simulink model "sldemo_fuelsys"  (R2022a)
settings: Solver=ode45  StartTime=0  StopTime=2000  FixedStep=0.001  RelTol=1e-5  AbsTol=1e-6
PostLoadFcn:
  | sldemo_fuelsys_data(bdroot,'initialize_data','orig','float');
model workspace (MAT data in the model file):
  PressEst = [0.806253176324 0.553142316929 0.37151500209 0.277667903103 0.220198954207 0.181288665766 0.153200000489 0.115431020872 0.0913067476324 0.0746519188607 0.0625231108324 0.0533383634277 ... (306 elements, 18x17)]
  PressVect = [0.05 0.1 0.15 0.2 0.25 0.3 0.35 0.4 0.45 0.5 0.55 0.6 0.65 0.7 0.75 0.8 0.85 0.9 0.95]
  PumpCon = [-0.0556348 -0.0022828 0.0256932 0.0435188 0.0562692 0.0661194857143 0.0741572 0.08697 0.0972452 0.106070342857 0.1139892 0.121303866667 ... (342 elements, 18x19)]
  RampRateKiX = [100 200 300 400 500 600]
  RampRateKiY = [0 0.2 0.4 0.6 0.8 1]
  RampRateKiZ = [0.012  0.024  0.036  0.048  0.06  0.072; 0.024  0.048  0.072  0.096  0.12  0.144; 0.036  0.072  0.108  0.144  0.18  0.216; 0.048  0.096  0.144  0.192  0.24  0.288; 0.06  0.12  0.18  0.24  0.3  0.36; 0.072  0.144  0.216  0.288  0.36  0.432]
  SpeedEst = [471.837839721 550.80940091 777.559313277 1080.9243499 1418.36795322 1769.7468768 2125.37309264 2480.20345067 2831.37796793 3177.14006959 3516.32917143 4064.90417867 ... (323 elements, 17x19)]
  SpeedVect = [50 75 100 125 150 175 200 250 300 350 400 450 500 600 700 800 900 1000]
  ThrotEst = [0 0 0 0 0 0 0 0 0 0 0 0 ... (342 elements, 18x19)]
  ThrotVect = [0 3 6 9 12 15 18 21 24 27 30 35 46 57 68 79 90]
  ego_sw = 1
  engine_speed = 300
  hys = 25
  map_sw = 1
  max_ego = 1.2
  max_press = 0.95
  max_speed = 628
  max_throt = 90
  min_press = 0.05
  min_speed = 50
  min_throt = 3
  speed_sw = 1
  st_range = 0.0001
  throttle_sw = 1
  zero_thresh = 250
undefined symbols (not defined in the file or in its folder): DiscIntNeverNeededParam, sld_FuelModes, sldvsubsys
libraries: simulink x4, simulink_extras x1
(part 1 of 2)
CloseFcn:
  | clear EngSensors u8En* s16En* sldemo_fuelsys_output
Description:
  | This is a model of a fuel control system where Stateflow(R) is used to handle the fault management of the system.
  | The system contains four separate sensors: a throttle sensor, a speed sensor, an oxygen sensor, and a pressure sensor.
  | Each of these sensors is represented by a parallel state in Stateflow.  Each parallel state contains two substates, a
  | normal state and a failed state (the exception being the oxygen sensor, which also contains a warmup state).
  | 
  | If any of the sensor readings is outside an acceptable range, then a fault is registered in Stateflow, and the
  | substate of the corresponding subsystem transitions to the failed state.  If a subsystem recovers, it can
  | transition back to the normal state.  The number of failures in the system at any given time is represented
  | in the Fail parallel state.
  | 
  | The last parallel state in the Stateflow chart is called Fueling_Mode.  This state regulates the oxygen to
  | fuel mixture ratio.  If a failure is detected, then the oxygen to fuel ratio is increased.  If multiple failures
  | are detected, then the fuel system is disabled until there are no longer multiple failures in the system.
settings Model: ModifiedByFormat=The MathWorks Inc.  ExtModeTrigMode=oneshot  ExtModeArmWhenConnect=off  Creator=The MathWorks, Inc.  LastModifiedBy=The MathWorks Inc.
settings SolverCC: AutoScaleAbsTol=off  AlgebraicLoopSolver=TrustRegion  MaxZcPerStep=1
settings DataIOCC: SaveFormat=StructureWithTime  SaveOutput=off  SaveTime=off  ReturnWorkspaceOutputs=off  SignalLoggingName=sldemo_fuelsys_output
settings OptimizationCC: DefaultParameterBehavior=Inlined  UseDivisionForNetSlopeComputation=UseDivisionForReciprocalsOfIntegersOnly  InlineInvariantSignals=on  EnhancedBackFolding=on  StrengthReduction=on  BooleansAsBitfields=on  PassReuseOutputArgsAs=Individual arguments  ExpressionDepthLimit=2147483647  ZeroExternalMemoryAtStartup=off  ZeroInternalMemoryAtStartup=off  NoFixptDivByZeroProtection=on  EfficientFloat2IntCast=on  LifeSpan=1  EfficientTunableParamExpr=on
settings DebuggingCC: SignalInfNanChecking=error  SaveWithParameterizedLinksMsg=none  UnderspecifiedInitializationDetection=Classic  CheckExecutionContextPreStartOutputMsg=on  IntegerOverflowMsg=none  ParameterDowncastMsg=warning  ParameterOverflowMsg=none  ParameterPrecisionLossMsg=none  UnderSpecifiedDataTypeMsg=warning  FcnCallInpInsideContextMsg=warning  UnconnectedInputMsg=warning  UnconnectedOutputMsg=warning  UnconnectedLineMsg=warning  UniqueDataStoreMsg=error  BusObjectLabelMismatch=error  AllowSymbolicDim=off  StateNameClashWarn=warning  StrictBusMsg=ErrorOnBusTreatedAsVector  SFUnexpectedBacktrackingDiag=warning  SFNoUnconditionalDefaultTransitionDiag=warning  SFExecutionAtInitializationDiag=none  SFMachineParentedDataDiag=warning  IntegerSaturationMsg=none  ArithmeticOperatorsInVariantConditions=warning
settings HardwareCC: ProdBitPerPointer=32  ProdBitPerSizeT=32  ProdBitPerPtrDiffT=32  ProdLargestAtomicFloat=None  ProdWordSize=32  ProdHWDeviceType=Specified
settings ModelReferenceCC: PropagateSignalLabelsOutOfModel=off
settings SFSimCC: SimUseLocalCustomCode=off  SimParseCustomCode=off  MATLABDynamicMemAlloc=off  CustomCodeUndefinedFunction=UseInterfaceOnly
settings RTWCC: Description=Real-Time Workshop Embedded Coder  SystemTargetFile=ert.tlc  TemplateMakefile=ert_default_tmf  GenerateReport=on  RTWVerbose=off  RTWUseLocalCustomCode=off  IncludeHyperlinkInReport=on  LaunchReport=on  GenerateTraceInfo=on  GenerateTraceReport=on  GenerateTraceReportSl=on  GenerateTraceReportSf=on  GenerateTraceReportEml=on  DLArmComputeVersion=19.05
settings CodeAppCC: ForceParamTrailComments=on  IgnoreCustomStorageClasses=off  IgnoreTestpoints=on  SimulinkDataObjDesc=on  SFDataObjDesc=on  CustomSymbolStrGlobalVar=rt$N$M  CustomSymbolStrType=$N$M  CustomSymbolStrFcn=$N$M$F  CustomSymbolStrModelFcn=$N  CustomSymbolStrMacro=$N$M  InsertBlockDesc=on  StateflowObjectComments=on  InternalIdentifier=Classic  ReqsInCode=on
settings ERTTargetCC: MultiwordLength=2048  GenerateSampleERTMain=on  IncludeMdlTerminateFcn=off  SupportAbsoluteTime=off  SupportNonFinite=off  SupportComplex=off  InlinedParameterPlacement=NonHierarchical  ERTCustomFileTemplate=example_file_process.tlc  ConvertIfToSwitch=off  SuppressUnreachableDefaultCases=off
settings ConfigComp: CovScope=Subsystem  CovPath=/fuel_rate_control/control_logic  CovMetricSettings=dw  CovSaveCumulativeToWorkspaceVar=on  CovSaveSingleToWorkspaceVar=on  CovExternalEMLEnable=off  CovSFcnEnable=off

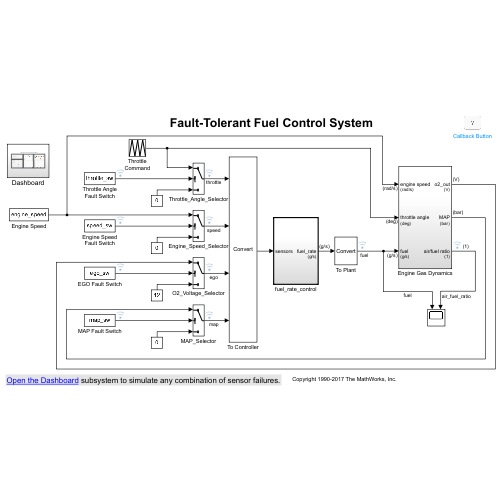
[thumbnail: Simulink's stored preview of the top-level diagram]
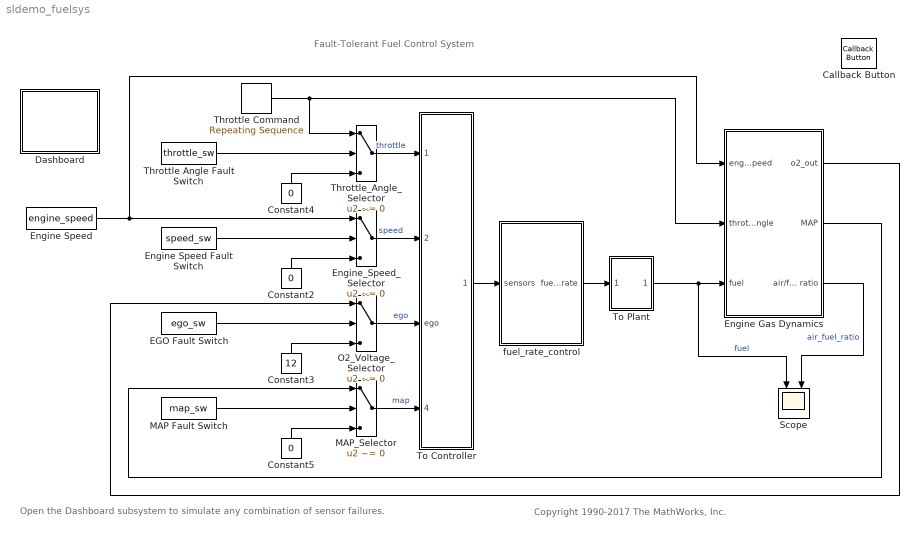
== system sldemo_fuelsys ==
  note: Fault-Tolerant Fuel Control System
  note: Copyright 1990-2017 The MathWorks, Inc.
  note: Open the Dashboard subsystem to simulate any combination of sensor failures.
  Callback Button : CallbackButton  ButtonText=?
      settings: ClickFcn=showExample('simulink_automotive/ModelingAFaultTolerantFuelControlSystemExample')
  Constant2 : Constant  Value=0
  Constant3 : Constant  Value=12
  Constant4 : Constant  Value=0
  Constant5 : Constant  Value=0
  Dashboard : Subsystem
  EGO Fault Switch : Constant  Value=ego_sw
  Engine Gas Dynamics : Subsystem
  Engine Speed : Constant  Value=engine_speed  SampleTime=[0,1]
  Engine Speed Fault Switch : Constant  Value=speed_sw
  Engine_Speed_Selector : Switch  Criteria=u2 ~= 0  Threshold=1  SaturateOnIntegerOverflow=off  InputSameDT=off
  MAP Fault Switch : Constant  Value=map_sw
  MAP_Selector : Switch  Criteria=u2 ~= 0  Threshold=1  SaturateOnIntegerOverflow=off  InputSameDT=off
  O2_Voltage_Selector : Switch  Criteria=u2 ~= 0  Threshold=1  SaturateOnIntegerOverflow=off  InputSameDT=off
  Scope : Scope  NumInputPorts=2
  Throttle Command : simulink/Sources/Repeating Sequence  rep_seq_t=[0 2 4]  rep_seq_y=[10 20 10]
  Throttle Angle Fault Switch : Constant  Value=throttle_sw
  Throttle_Angle_Selector : Switch  Criteria=u2 ~= 0  Threshold=1  SaturateOnIntegerOverflow=off  InputSameDT=off
  To Controller : Subsystem
      mask Display: fprintf('Convert')
  To Plant : Subsystem
      mask Display: fprintf('Convert')
  fuel_rate_control : Subsystem  Tag=FuelRateControl  TreatAsAtomicUnit=on
  wires:
  fuel_rate_control/1(fuel_rate) -> To Plant/1(In1)
  To Plant/1(Out1) -> Scope/1, Engine Gas Dynamics/3(fuel)  "fuel"
  To Controller/1(sensors) -> fuel_rate_control/1(sensors)
  Throttle_Angle_Selector/1 -> To Controller/1(throttle)  "throttle"
  Engine_Speed_Selector/1 -> To Controller/2(speed)  "speed"
  O2_Voltage_Selector/1 -> To Controller/3(ego)  "ego"
  MAP_Selector/1 -> To Controller/4(map)  "map"
  Constant4/1 -> Throttle_Angle_Selector/3
  Throttle Command/1 -> Throttle_Angle_Selector/1, Engine Gas Dynamics/2(throttle angle)
  Throttle Angle Fault Switch/1 -> Throttle_Angle_Selector/2
  Engine Speed Fault Switch/1 -> Engine_Speed_Selector/2
  Engine Speed/1 -> Engine Gas Dynamics/1(engine speed), Engine_Speed_Selector/1
  Constant2/1 -> Engine_Speed_Selector/3
  Constant3/1 -> O2_Voltage_Selector/3
  Engine Gas Dynamics/1(o2_out) -> O2_Voltage_Selector/1
  EGO Fault Switch/1 -> O2_Voltage_Selector/2
  MAP Fault Switch/1 -> MAP_Selector/2
  Engine Gas Dynamics/2(MAP) -> MAP_Selector/1
  Constant5/1 -> MAP_Selector/3
  Engine Gas Dynamics/3(air/fuel ratio) -> Scope/2  "air_fuel_ratio"

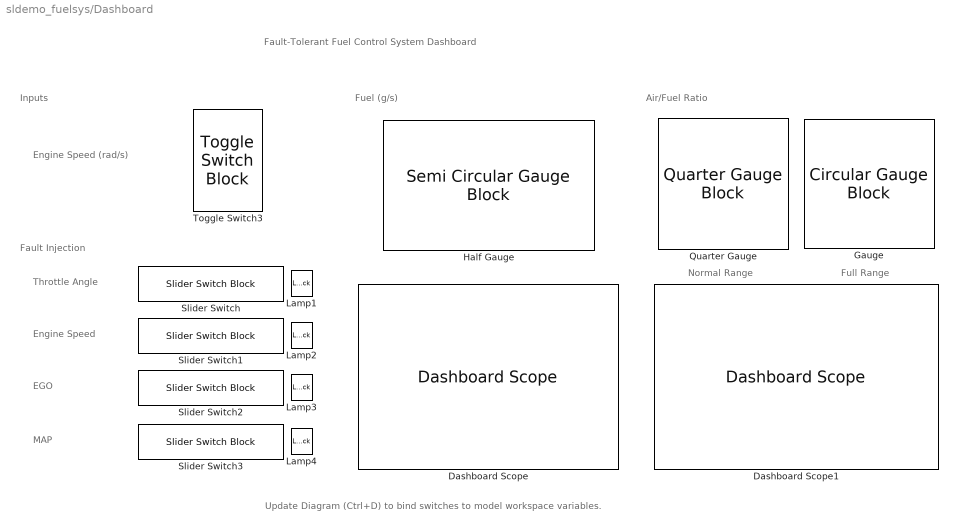
== system sldemo_fuelsys/Dashboard ==
  note: Inputs
  note: Fault Injection
  note: Air/Fuel Ratio
  note: Fuel (g/s)
  note: Throttle Angle
  note: Engine Speed
  note: EGO
  note: Fault-Tolerant Fuel Control System Dashboard
  note: MAP
  note: Engine Speed (rad/s)
  note: Normal Range
  note: Full Range
  note: Update Diagram (Ctrl+D) to bind switches to model workspace variables.
  Dashboard Scope : DashboardScope  TimeSpan=500  Ymin=0  LegendPosition=Hide  ScaleAtStop=off
  Dashboard Scope1 : DashboardScope  TimeSpan=500  Ymin=0  Ymax=400  LegendPosition=Hide  ScaleAtStop=off
  Gauge : CircularGaugeBlock  LabelPosition=Hide  ScaleMax=400
  Half Gauge : SemiCircularGaugeBlock  LabelPosition=Hide  ScaleMax=3
  Lamp{1..4} (4 alike) : LampBlock  LabelPosition=Hide
  Quarter Gauge : QuarterGaugeBlock  LabelPosition=Hide  ScaleMax=20
  Slider Switch{,1..3} (4 alike) : SliderSwitchBlock  LabelPosition=Hide
      settings: Values={{'NORMAL', 'FAIL'}, [1 0]}
  Toggle Switch3 : ToggleSwitchBlock  LabelPosition=Hide
      settings: Values={{'700', '300'}, [700 300]}

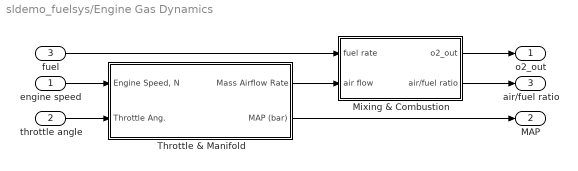
== system sldemo_fuelsys/Engine Gas Dynamics ==
  engine speed : Inport  Unit=rad/s
  throttle angle : Inport  Port=2  Unit=deg
  fuel : Inport  Port=3  Unit=g/s
  Mixing & Combustion : Subsystem
  Throttle & Manifold : Subsystem
  o2_out : Outport  Unit=V  VectorParamsAs1DForOutWhenUnconnected=off
  MAP : Outport  Port=2  Unit=bar  VectorParamsAs1DForOutWhenUnconnected=off
  air/fuel ratio : Outport  Port=3  Unit=1  VectorParamsAs1DForOutWhenUnconnected=off
  wires:
  Throttle & Manifold/1(Mass Airflow Rate) -> Mixing & Combustion/2(air flow)
  fuel/1 -> Mixing & Combustion/1(fuel rate)
  engine speed/1 -> Throttle & Manifold/1("Engine Speed, N")
  throttle angle/1 -> Throttle & Manifold/2(Throttle Ang.)
  Mixing & Combustion/2(air/fuel ratio) -> air/fuel ratio/1
  Throttle & Manifold/2(MAP (bar)) -> MAP/1
  Mixing & Combustion/1(o2_out) -> o2_out/1

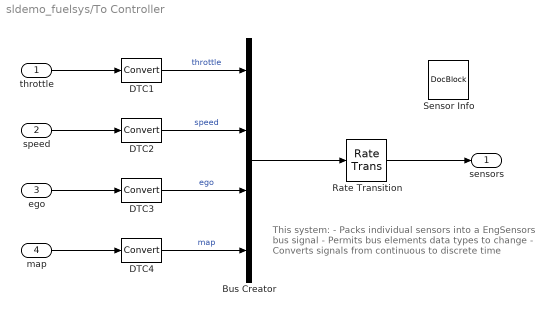
== system sldemo_fuelsys/To Controller ==
  note: This system:
      | - Packs individual sensors into a EngSensors bus signal
      | - Permits bus elements data types to change
      | - Converts signals from continuous to discrete time
  throttle : Inport
  speed : Inport  Port=2
  ego : Inport  Port=3
  map : Inport  Port=4
  Bus Creator : BusCreator  Inputs=4  OutDataTypeStr=Bus: EngSensors  NonVirtualBus=on
  DTC{1..4} (4 alike) : DataTypeConversion  SampleTime=[0 1]  SaturateOnIntegerOverflow=off  RndMeth=Floor
  Rate Transition : RateTransition  OutPortSampleTime=0.01
  Sensor Info : simulink/Model-Wide Utilities/DocBlock  DocumentType=Text
      content=|
      | Measurement Descriptions
      | ========================
      |
      | Throttle Angle (degrees):
      | min=3, max=90, precision=0.1
      |
      | Engine Speed (radians/sec.):
      | min=0, max=620, precision=.1
      |
      | Ego Sensor (volts):
      | min=0, max=12, precision=.05
      |
      | Manifold Pressure (bar):
      | min=0.001, max=1, precision=.001
  sensors : Outport  VectorParamsAs1DForOutWhenUnconnected=off
  wires:
  throttle/1 -> DTC1/1
  DTC1/1 -> Bus Creator/1  "throttle"
  speed/1 -> DTC2/1
  DTC2/1 -> Bus Creator/2  "speed"
  ego/1 -> DTC3/1
  DTC3/1 -> Bus Creator/3  "ego"
  map/1 -> DTC4/1
  DTC4/1 -> Bus Creator/4  "map"
  Bus Creator/1 -> Rate Transition/1
  Rate Transition/1 -> sensors/1

== system sldemo_fuelsys/To Plant ==
  note: This system:
      | - Permits upstream signal data type to change
      | - Converts signals from discrete to continuous time
  In1 : Inport
  DTC5 : DataTypeConversion  SaturateOnIntegerOverflow=off  RndMeth=Floor
  Rate Transition1 : RateTransition  Integrity=off  InitialCondition=1.6  OutPortSampleTime=0
  Out1 : Outport  VectorParamsAs1DForOutWhenUnconnected=off
  wires:
  DTC5/1 -> Rate Transition1/1
  In1/1 -> DTC5/1
  Rate Transition1/1 -> Out1/1

== system sldemo_fuelsys/fuel_rate_control ==
  note: Fuel Rate Control Subsystem
  sensors : Inport  OutDataTypeStr=Bus: EngSensors
  Bus Selector1 : BusSelector  OutputSignals=speed
  airflow_calc : Subsystem
  control_logic : Stateflow chart  Description=Stateflow diagram to determine control system operating mode  TreatAsAtomicUnit=on
  fuel_calc : Subsystem
  validate_sample_time : Subsystem  Tag=VerificationSubsystem  DisableCoverage=on  LoadFcn=sldvsubsys('check')  TreatAsAtomicUnit=on  SimViewingDevice=on  mask(VerificationSubsystem){}
      mask init:
      | sldvsubsys('maskInit');
      settings: CopyFcn=sldvsubsys('copy');  OpenFcn=open_system(gcb,'force');
      settings: PreSaveFcn=|
      | set_param(gcb,'SimViewingDevice','on');
      | sldvsubsys('check');
      mask Help: helpview(fullfile(docroot,'toolbox','sldv','sldv.map'),'verificationsubsystem')
      mask Display: image(imread('sldvicon_versubsys.png','BackGroundColor',[1 1 1]),'center');
  fuel_rate : Outport  Unit=g/s  VectorParamsAs1DForOutWhenUnconnected=off
  wires:
  fuel_calc/1(fuel_rate) -> fuel_rate/1
  airflow_calc/1(est_airflow) -> fuel_calc/1(est_airflow)
  sensors/1 -> control_logic/1(es_i), Bus Selector1/1
  control_logic/3(fuel_mode) -> airflow_calc/3(fuel_mode), fuel_calc/3(fuel_mode)
  control_logic/1(es_o) -> airflow_calc/1(sensors)
  control_logic/2(" O2_normal") -> airflow_calc/2(O2_normal)
  airflow_calc/2(fb_correction) -> fuel_calc/2(fb_correction)
  Bus Selector1/1 -> validate_sample_time/1(In1)  "<speed>"

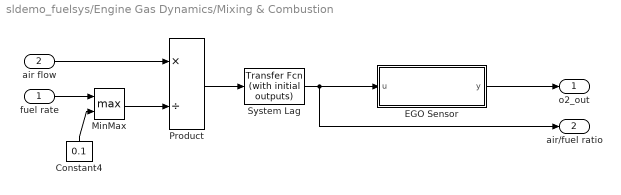
== system sldemo_fuelsys/Engine Gas Dynamics/Mixing & Combustion ==
  fuel rate : Inport  Unit=g/s
  air flow : Inport  Port=2  Unit=g/s
  Constant4 : Constant  Value=0.1
  EGO Sensor : MATLAB Function  TreatAsAtomicUnit=on
  MinMax : MinMax  Function=max  Inputs=2  InputSameDT=on  SaturateOnIntegerOverflow=on
  Product : Product  Inputs=*/  InputSameDT=on  RndMeth=Zero  SaturateOnIntegerOverflow=on  OutDataTypeStr=Inherit: Same as first input
  System Lag : simulink_extras/Additional Linear/Transfer Fcn (with initial outputs)  N=3  D=[1 3]  Y0=1/14.6  U0=1/14.6
  o2_out : Outport  Unit=V  VectorParamsAs1DForOutWhenUnconnected=off
  air/fuel ratio : Outport  Port=2  Unit=1  VectorParamsAs1DForOutWhenUnconnected=off
  wires:
  Constant4/1 -> MinMax/2
  fuel rate/1 -> MinMax/1
  MinMax/1 -> Product/2
  Product/1 -> System Lag/1
  System Lag/1 -> air/fuel ratio/1, EGO Sensor/1(u)
  EGO Sensor/1(y) -> o2_out/1
  air flow/1 -> Product/1

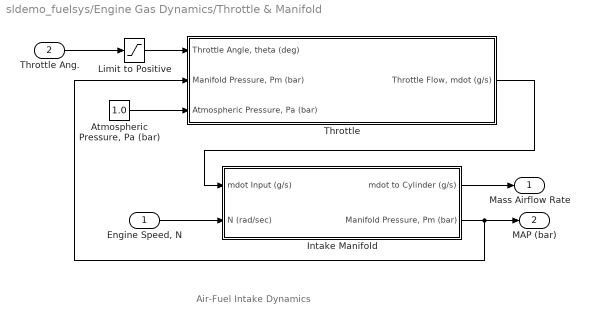
== system sldemo_fuelsys/Engine Gas Dynamics/Throttle & Manifold ==
  note: Air-Fuel Intake Dynamics
  "Engine Speed, N" : Inport  Unit=rad/s
  Throttle Ang. : Inport  Port=2  Unit=deg
  "Atmospheric Pressure, Pa (bar)" : Constant  Value=1.0
  Intake Manifold : Subsystem
  Limit to Positive : Saturate  UpperLimit=inf  LowerLimit=0
  Throttle : Subsystem
  Mass Airflow Rate : Outport  Unit=g/s  VectorParamsAs1DForOutWhenUnconnected=off
  MAP (bar) : Outport  Port=2  Unit=bar  VectorParamsAs1DForOutWhenUnconnected=off
  wires:
  Limit to Positive/1 -> Throttle/1("Throttle Angle, theta (deg)")
  Throttle Ang./1 -> Limit to Positive/1
  Throttle/1("Throttle Flow, mdot (g/s)") -> Intake Manifold/1(mdot Input (g/s))
  "Engine Speed, N"/1 -> Intake Manifold/2(N (rad/sec))
  Intake Manifold/1(mdot to Cylinder (g/s)) -> Mass Airflow Rate/1
  "Atmospheric Pressure, Pa (bar)"/1 -> Throttle/3("Atmospheric Pressure, Pa (bar) ")
  Intake Manifold/2("Manifold Pressure, Pm (bar)") -> Throttle/2("Manifold Pressure, Pm (bar)"), MAP (bar)/1

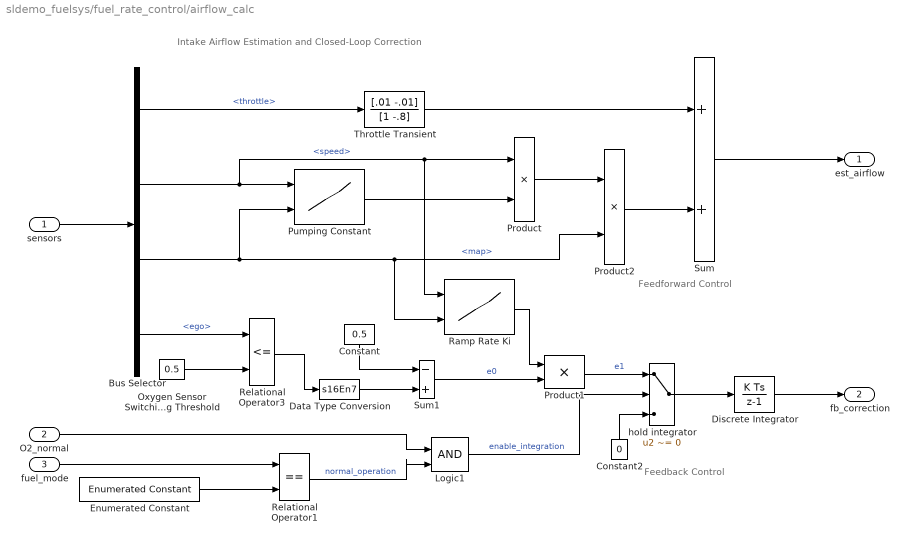
== system sldemo_fuelsys/fuel_rate_control/airflow_calc ==
  note: Intake Airflow Estimation and Closed-Loop Correction
  note: Feedback Control
  note: Feedforward Control
  sensors : Inport
  O2_normal : Inport  Port=2
  fuel_mode : Inport  Port=3
  Bus Selector : BusSelector  OutputSignals=throttle,speed,map,ego
  Constant : Constant  Value=0.5  OutDataTypeStr=s16En7
  Constant2 : Constant  Value=0  OutDataTypeStr=uint8
  Data Type Conversion : DataTypeConversion  OutDataTypeStr=s16En7  RndMeth=Simplest  SaturateOnIntegerOverflow=off
  Discrete Integrator : DiscreteIntegrator  SampleTime=-1  OutDataTypeStr=s16En15  RndMeth=Simplest  ICPrevOutput=DiscIntNeverNeededParam  ICPrevScaledInput=DiscIntNeverNeededParam
  Enumerated Constant : simulink/Sources/Enumerated Constant  OutDataTypeStr=Enum: sld_FuelModes  Value=sld_FuelModes.LOW  SampleTime=.01
  Logic1 : Logic  IconShape=distinctive  AllPortsSameDT=off  OutDataTypeStr=boolean
  Oxygen Sensor Switching Threshold : Constant  Value=0.5  OutDataTypeStr=s16En7
  Product : Product  OutDataTypeStr=s16En7  RndMeth=Simplest
  Product1 : Product  OutDataTypeStr=s16En15  RndMeth=Simplest
  Product2 : Product  OutDataTypeStr=s16En7  RndMeth=Simplest
  Pumping Constant : Lookup_n-D  LookupTableObject=''  BreakpointsForDimension1=SpeedVect  BreakpointsForDimension2=PressVect  IndexSearchMethod=Linear search  Table=PumpCon  ExtrapMethod=Clip  UseLastTableValue=on  OutDataTypeStr=s16En15  RndMeth=Simplest  InputSameDT=off
      settings: InputPortMap=u0,u1
  Ramp Rate Ki : Lookup_n-D  LookupTableObject=''  BreakpointsForDimension1=RampRateKiX  BreakpointsForDimension2=RampRateKiY  IndexSearchMethod=Linear search  Table=RampRateKiZ  ExtrapMethod=Clip  UseLastTableValue=on  OutDataTypeStr=s16En15  RndMeth=Simplest  InputSameDT=off
      settings: InputPortMap=u0,u1
  Relational Operator1 : RelationalOperator  Operator===  OutDataTypeStr=boolean
  Relational Operator3 : RelationalOperator  Operator=<=  OutDataTypeStr=boolean  InputSameDT=off
  Sum : Sum  Inputs=2  OutDataTypeStr=s16En7  RndMeth=Simplest
  Sum1 : Sum  Inputs=-+  OutDataTypeStr=s16En15  RndMeth=Simplest
  Throttle Transient : DiscreteFilter  Numerator=[.01 -.01]  Denominator=[1 -.8]  a0EqualsOne=on  OutDataTypeStr=s16En7  RndMeth=Simplest
  hold integrator : Switch  Criteria=u2 ~= 0  Threshold=1  OutDataTypeStr=s16En15  RndMeth=Simplest  SaturateOnIntegerOverflow=off  InputSameDT=off
  est_airflow : Outport  Unit=g/s  VectorParamsAs1DForOutWhenUnconnected=off
  fb_correction : Outport  Port=2  VectorParamsAs1DForOutWhenUnconnected=off
  wires:
  Discrete Integrator/1 -> fb_correction/1
  sensors/1 -> Bus Selector/1
  Pumping Constant/1 -> Product/2
  Bus Selector/2 -> Product/1, Ramp Rate Ki/1, Pumping Constant/1  "<speed>"
  Throttle Transient/1 -> Sum/1
  Sum/1 -> est_airflow/1
  Bus Selector/1 -> Throttle Transient/1  "<throttle>"
  Relational Operator1/1 -> Logic1/2  "normal_operation"
  Oxygen Sensor Switching Threshold/1 -> Relational Operator3/2
  Constant/1 -> Sum1/1
  Ramp Rate Ki/1 -> Product1/1
  Constant2/1 -> hold integrator/3
  Product1/1 -> hold integrator/1  "e1"
  hold integrator/1 -> Discrete Integrator/1
  Logic1/1 -> hold integrator/2  "enable_integration"
  Sum1/1 -> Product1/2  "e0"
  Relational Operator3/1 -> Data Type Conversion/1
  Data Type Conversion/1 -> Sum1/2
  Bus Selector/3 -> Product2/2, Ramp Rate Ki/2, Pumping Constant/2  "<map>"
  Bus Selector/4 -> Relational Operator3/1  "<ego>"
  Product/1 -> Product2/1
  Product2/1 -> Sum/2
  O2_normal/1 -> Logic1/1
  Enumerated Constant/1 -> Relational Operator1/2
  fuel_mode/1 -> Relational Operator1/1

== system sldemo_fuelsys/fuel_rate_control/control_logic/Pressure.map_estimate ==
  note: MAP Estimation
  speed : Inport  OutDataTypeStr=s16En3
  throttle : Inport  Port=2  OutDataTypeStr=s16En3
  f : TriggerPort  TriggerType=function-call  VariantControl=Variant
      settings: CopyFcn=Stateflow.SLINSF.SimulinkMan.removeBlockPreDeleteFcn  PreDeleteFcn=Stateflow.SLINSF.SimulinkMan.unsafePredeleteFcn
  Pressure Estimation : Lookup_n-D  LookupTableObject=''  BreakpointsForDimension1=SpeedVect  BreakpointsForDimension2=ThrotVect  IndexSearchMethod=Linear search  Table=PressEst  ExtrapMethod=Clip  UseLastTableValue=on  OutDataTypeStr=u8En7  RndMeth=Simplest  InputSameDT=off
      settings: InputPortMap=u0,u1
  map : Outport  VectorParamsAs1DForOutWhenUnconnected=off
  wires:
  speed/1 -> Pressure Estimation/1
  throttle/1 -> Pressure Estimation/2
  Pressure Estimation/1 -> map/1

== system sldemo_fuelsys/fuel_rate_control/control_logic/Speed.speed_estimate ==
  note: Speed Estimation
  throttle : Inport  OutDataTypeStr=s16En3
  map : Inport  Port=2  OutDataTypeStr=u8En7
  f : TriggerPort  TriggerType=function-call  VariantControl=Variant
      settings: CopyFcn=Stateflow.SLINSF.SimulinkMan.removeBlockPreDeleteFcn  PreDeleteFcn=Stateflow.SLINSF.SimulinkMan.unsafePredeleteFcn
  Saturation : Saturate  UpperLimit=max_speed  LowerLimit=0  OutDataTypeStr=s16En3
  Speed Estimation : Lookup_n-D  LookupTableObject=''  BreakpointsForDimension1=ThrotVect  BreakpointsForDimension2=PressVect  IndexSearchMethod=Linear search  Table=SpeedEst  ExtrapMethod=Clip  UseLastTableValue=on  OutDataTypeStr=s16En3  RndMeth=Simplest  InputSameDT=off
      settings: InputPortMap=u0,u1
  speed : Outport  VectorParamsAs1DForOutWhenUnconnected=off
  wires:
  Speed Estimation/1 -> Saturation/1
  throttle/1 -> Speed Estimation/1
  map/1 -> Speed Estimation/2
  Saturation/1 -> speed/1

== system sldemo_fuelsys/fuel_rate_control/control_logic/Throttle.throttle_estimate ==
  note: Throttle Estimation
  speed : Inport  OutDataTypeStr=s16En3
  map : Inport  Port=2  OutDataTypeStr=u8En7
  f : TriggerPort  TriggerType=function-call  VariantControl=Variant
      settings: CopyFcn=Stateflow.SLINSF.SimulinkMan.removeBlockPreDeleteFcn  PreDeleteFcn=Stateflow.SLINSF.SimulinkMan.unsafePredeleteFcn
  Throttle Estimation : Lookup_n-D  LookupTableObject=''  BreakpointsForDimension1=SpeedVect  BreakpointsForDimension2=PressVect  IndexSearchMethod=Linear search  Table=ThrotEst  ExtrapMethod=Clip  UseLastTableValue=on  OutDataTypeStr=s16En7  RndMeth=Simplest  InputSameDT=off
      settings: InputPortMap=u0,u1
  throttle : Outport  VectorParamsAs1DForOutWhenUnconnected=off
  wires:
  speed/1 -> Throttle Estimation/1
  map/1 -> Throttle Estimation/2
  Throttle Estimation/1 -> throttle/1

== system sldemo_fuelsys/fuel_rate_control/fuel_calc ==
  note: Fuel Rate Calculation
  est_airflow : Inport  Unit=g/s
  fb_correction : Inport  Port=2
  fuel_mode : Inport  Port=3
  feedforward_fuel_rate : Subsystem
  switchable_compensation : Subsystem
  fuel_rate : Outport  Unit=g/s  VectorParamsAs1DForOutWhenUnconnected=off
  wires:
  est_airflow/1 -> feedforward_fuel_rate/1(est_airflow)
  fuel_mode/1 -> feedforward_fuel_rate/2(fuel_mode), switchable_compensation/2(fuel_mode)
  switchable_compensation/1(fuel_rate) -> fuel_rate/1
  fb_correction/1 -> switchable_compensation/3(fb_correction)
  feedforward_fuel_rate/1(ff_fuel_rate) -> switchable_compensation/1(ff_fuel_rate)

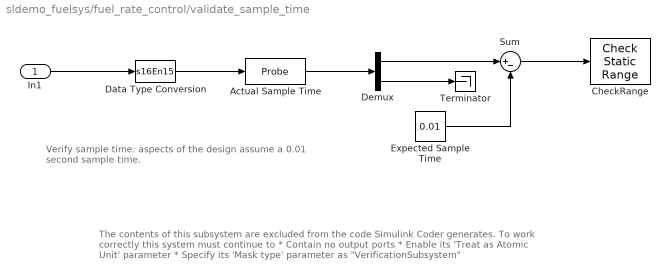
== system sldemo_fuelsys/fuel_rate_control/validate_sample_time ==
  note: The contents of this subsystem are excluded from the code Simulink Coder generates.
      |
      | To work correctly this system must continue to
      | * Contain no output ports
      | * Enable its 'Treat as Atomic Unit' parameter
      | * Specify its 'Mask type' parameter as "VerificationSubsystem"
  note: Verify sample time: aspects of the design
      | assume a 0.01 second sample time.
  In1 : Inport
  Actual Sample Time : Probe  ProbeWidth=off  ProbeComplexSignal=off  ProbeSampleTimeDataType=Same as input
  CheckRange : simulink/Model Verification/Check  Static Range  Description=-st_range < u < st_range  max=st_range  max_included=off  min=-st_range  min_included=off  enabled=on  stopWhenAssertionFail=on  export=off  icon=graphic
      settings: SourceProductBaseCode=SL
  Data Type Conversion : DataTypeConversion  OutDataTypeStr=s16En15  SaturateOnIntegerOverflow=off  RndMeth=Floor
  Demux : Demux  Outputs=2
  Expected Sample Time : Constant  Value=0.01  OutDataTypeStr=s16En15
  Sum : Sum  Inputs=|+-  OutDataTypeStr=Inherit: Same as first input
  Terminator : Terminator
  wires:
  Actual Sample Time/1 -> Demux/1
  In1/1 -> Data Type Conversion/1
  Demux/2 -> Terminator/1
  Demux/1 -> Sum/1
  Expected Sample Time/1 -> Sum/2
  Sum/1 -> CheckRange/1
  Data Type Conversion/1 -> Actual Sample Time/1

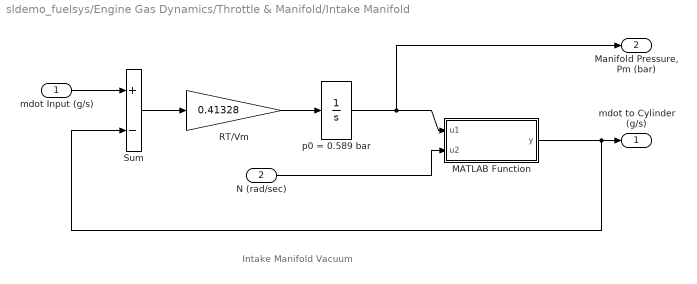
== system sldemo_fuelsys/Engine Gas Dynamics/Throttle & Manifold/Intake Manifold ==
  note: Intake Manifold Vacuum
  mdot Input (g/s) : Inport  Unit=g/s
  N (rad/sec) : Inport  Port=2  Unit=rad/s
  MATLAB Function : MATLAB Function  TreatAsAtomicUnit=on
  RT/Vm : Gain  Gain=0.41328  SaturateOnIntegerOverflow=on  OutDataTypeStr=Inherit: Same as input  ParamDataTypeStr=Inherit: Same as input
  Sum : Sum  Inputs=+-  InputSameDT=on  SaturateOnIntegerOverflow=on  OutDataTypeStr=Inherit: Same as first input
  p0 = 0.589 bar : Integrator  InitialCondition=.589
  mdot to Cylinder (g/s) : Outport  Unit=g/s  VectorParamsAs1DForOutWhenUnconnected=off
  "Manifold Pressure, Pm (bar)" : Outport  Port=2  Unit=bar  VectorParamsAs1DForOutWhenUnconnected=off
  wires:
  mdot Input (g/s)/1 -> Sum/1
  RT/Vm/1 -> p0 = 0.589 bar/1
  N (rad/sec)/1 -> MATLAB Function/2(u2)
  p0 = 0.589 bar/1 -> "Manifold Pressure, Pm (bar)"/1, MATLAB Function/1(u1)
  Sum/1 -> RT/Vm/1
  MATLAB Function/1(y) -> mdot to Cylinder (g/s)/1, Sum/2

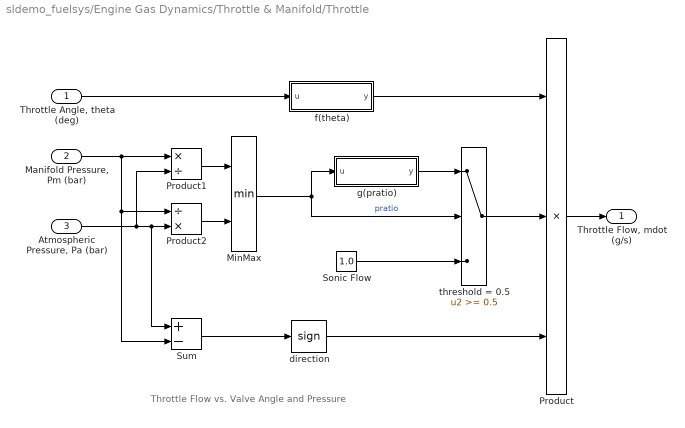
== system sldemo_fuelsys/Engine Gas Dynamics/Throttle & Manifold/Throttle ==
  note: Throttle Flow vs. Valve Angle and Pressure
  "Throttle Angle, theta (deg)" : Inport  Unit=deg
  "Manifold Pressure, Pm (bar)" : Inport  Port=2  Unit=bar
  "Atmospheric Pressure, Pa (bar) " : Inport  Port=3  Unit=bar
  MinMax : MinMax  Inputs=2  InputSameDT=on  SaturateOnIntegerOverflow=on
  Product : Product  Inputs=3  InputSameDT=on  RndMeth=Zero  SaturateOnIntegerOverflow=on  OutDataTypeStr=Inherit: Same as first input
  Product1 : Product  Inputs=*/  InputSameDT=on  RndMeth=Zero  SaturateOnIntegerOverflow=on  OutDataTypeStr=Inherit: Same as first input
  Product2 : Product  Inputs=/*  InputSameDT=on  RndMeth=Zero  SaturateOnIntegerOverflow=on  OutDataTypeStr=Inherit: Same as first input
  "Sonic Flow " : Constant  Value=1.0
  Sum : Sum  Inputs=+-  InputSameDT=on  SaturateOnIntegerOverflow=on  OutDataTypeStr=Inherit: Same as first input
  direction : Signum
  f(theta) : MATLAB Function  TreatAsAtomicUnit=on
  g(pratio) : MATLAB Function  TreatAsAtomicUnit=on
  threshold = 0.5 : Switch  Threshold=0.5
  "Throttle Flow, mdot (g/s)" : Outport  Unit=g/s  VectorParamsAs1DForOutWhenUnconnected=off
  wires:
  "Manifold Pressure, Pm (bar)"/1 -> Sum/2, Product2/1, Product1/1
  Product2/1 -> MinMax/2
  Product1/1 -> MinMax/1
  "Atmospheric Pressure, Pa (bar) "/1 -> Sum/1, Product2/2, Product1/2
  g(pratio)/1(y) -> threshold = 0.5/1
  "Sonic Flow "/1 -> threshold = 0.5/3
  threshold = 0.5/1 -> Product/2
  direction/1 -> Product/3
  Sum/1 -> direction/1
  MinMax/1 -> threshold = 0.5/2, g(pratio)/1(u)  "pratio"
  "Throttle Angle, theta (deg)"/1 -> f(theta)/1(u)
  Product/1 -> "Throttle Flow, mdot (g/s)"/1
  f(theta)/1(y) -> Product/1

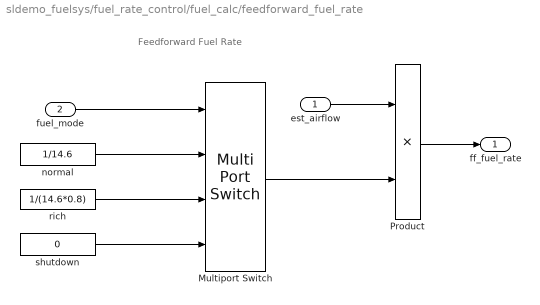
== system sldemo_fuelsys/fuel_rate_control/fuel_calc/feedforward_fuel_rate ==
  note: Feedforward Fuel Rate
  est_airflow : Inport
  fuel_mode : Inport  Port=2
  Multiport Switch : MultiPortSwitch  DataPortOrder=Specify indices  DataPortIndices={sld_FuelModes.LOW, sld_FuelModes.RICH, sld_FuelModes.DISABLED}  OutDataTypeStr=s16En7  RndMeth=Simplest  SaturateOnIntegerOverflow=off  InputSameDT=off
  Product : Product  OutDataTypeStr=s16En7  RndMeth=Simplest
  normal : Constant  Value=1/14.6  OutDataTypeStr=s16En7
  rich : Constant  Value=1/(14.6*0.8)  OutDataTypeStr=s16En7
  shutdown : Constant  Value=0  OutDataTypeStr=s16En7
  ff_fuel_rate : Outport  VectorParamsAs1DForOutWhenUnconnected=off
  wires:
  rich/1 -> Multiport Switch/3
  fuel_mode/1 -> Multiport Switch/1
  est_airflow/1 -> Product/1
  Product/1 -> ff_fuel_rate/1
  Multiport Switch/1 -> Product/2
  normal/1 -> Multiport Switch/2
  shutdown/1 -> Multiport Switch/4

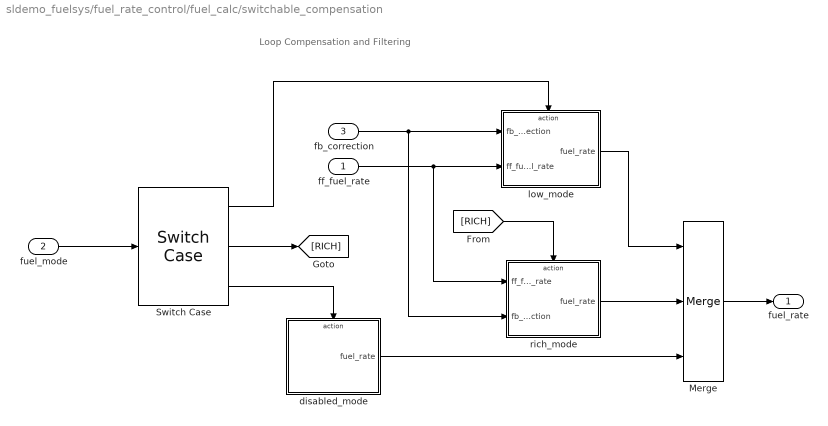
== system sldemo_fuelsys/fuel_rate_control/fuel_calc/switchable_compensation ==
  note: Loop Compensation and Filtering
  ff_fuel_rate : Inport
  fuel_mode : Inport  Port=2
  fb_correction : Inport  Port=3
  Merge : Merge  Inputs=3
  Switch Case : SwitchCase  CaseConditions={sld_FuelModes.LOW, sld_FuelModes.RICH}
  disabled_mode : Subsystem  TreatAsAtomicUnit=on
  low_mode : Subsystem  TreatAsAtomicUnit=on
  rich_mode : Subsystem  TreatAsAtomicUnit=on
  fuel_rate : Outport  VectorParamsAs1DForOutWhenUnconnected=off
  wires:
  fuel_mode/1 -> Switch Case/1
  ff_fuel_rate/1 -> rich_mode/1(ff_fuel_rate), low_mode/2(ff_fuel_rate)
  fb_correction/1 -> rich_mode/2(fb_correction), low_mode/1(fb_correction)
  Switch Case/1 -> low_mode/Action
  Switch Case/2 -> [RICH]
  [RICH] -> rich_mode/Action
  Switch Case/3 -> disabled_mode/Action
  rich_mode/1(fuel_rate) -> Merge/2
  disabled_mode/1(fuel_rate) -> Merge/3
  low_mode/1(fuel_rate) -> Merge/1
  Merge/1 -> fuel_rate/1

== system sldemo_fuelsys/fuel_rate_control/fuel_calc/switchable_compensation/disabled_mode ==
  note: Disabled Mode Fuel Mode
  Action Port : ActionPort  ActionPortLabel=default: { }
  shutoff : Constant  Value=0  OutDataTypeStr=Inherit: Inherit via back propagation
  fuel_rate : Outport  InitialOutput=0  VectorParamsAs1DForOutWhenUnconnected=off
  wires:
  shutoff/1 -> fuel_rate/1

== system sldemo_fuelsys/fuel_rate_control/fuel_calc/switchable_compensation/low_mode ==
  note: Low Mode Fuel Mode
  fb_correction : Inport
  ff_fuel_rate : Inport  Port=2
  Action Port : ActionPort  ActionPortLabel=case: { }
  Discrete Filter : DiscreteFilter  Numerator=[8.7696 -8.5104]  Denominator=[1 -0.7408]  a0EqualsOne=on  RndMeth=Simplest  OutDataTypeStr=Inherit: Same as input
  Sum3 : Sum  OutDataTypeStr=s16En7  RndMeth=Simplest
  fuel_rate : Outport  InitialOutput=0  VectorParamsAs1DForOutWhenUnconnected=off
  wires:
  ff_fuel_rate/1 -> Sum3/2
  Discrete Filter/1 -> Sum3/1
  Sum3/1 -> fuel_rate/1
  fb_correction/1 -> Discrete Filter/1

== system sldemo_fuelsys/fuel_rate_control/fuel_calc/switchable_compensation/rich_mode ==
  note: Rich Mode Fuel Mode
  ff_fuel_rate : Inport
  fb_correction : Inport  Port=2
  Action Port : ActionPort  ActionPortLabel=case: { }
  Discrete Filter : DiscreteFilter  Numerator=[0 0.2592]  Denominator=[1 -0.7408]  a0EqualsOne=on  RndMeth=Simplest  OutDataTypeStr=Inherit: Same as input
  Sum2 : Sum  OutDataTypeStr=s16En7  RndMeth=Simplest
  fuel_rate : Outport  InitialOutput=0  VectorParamsAs1DForOutWhenUnconnected=off
  wires:
  fb_correction/1 -> Sum2/2
  ff_fuel_rate/1 -> Sum2/1
  Sum2/1 -> Discrete Filter/1
  Discrete Filter/1 -> fuel_rate/1
